simulink model "H_Full_Bridge_Inverter"  (R2023b)
settings: Solver=FixedStepDiscrete  StartTime=0.0  StopTime=0.1  FixedStep=10e-6  RelTol=1e-3
libraries: spsIGBTDiodeLib x4, simulink x1, spsCurrentMeasurementLib x1, spsDCVoltageSourceLib x1, spsSeriesRLCBranchLib x1, spsVoltageMeasurementLib x1, sps_lib x1
settings Model: Creator=aoni5  LastModifiedBy=aoni5

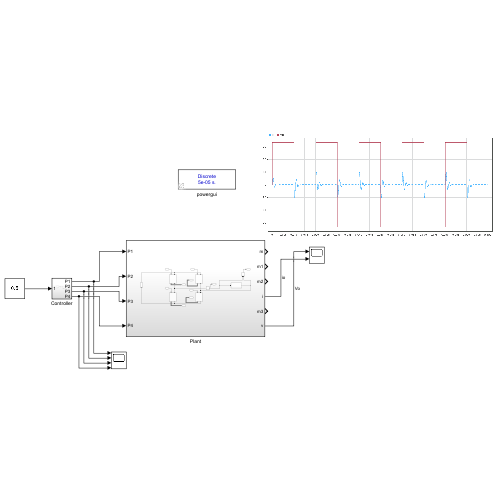
[thumbnail: Simulink's stored preview of the top-level diagram]
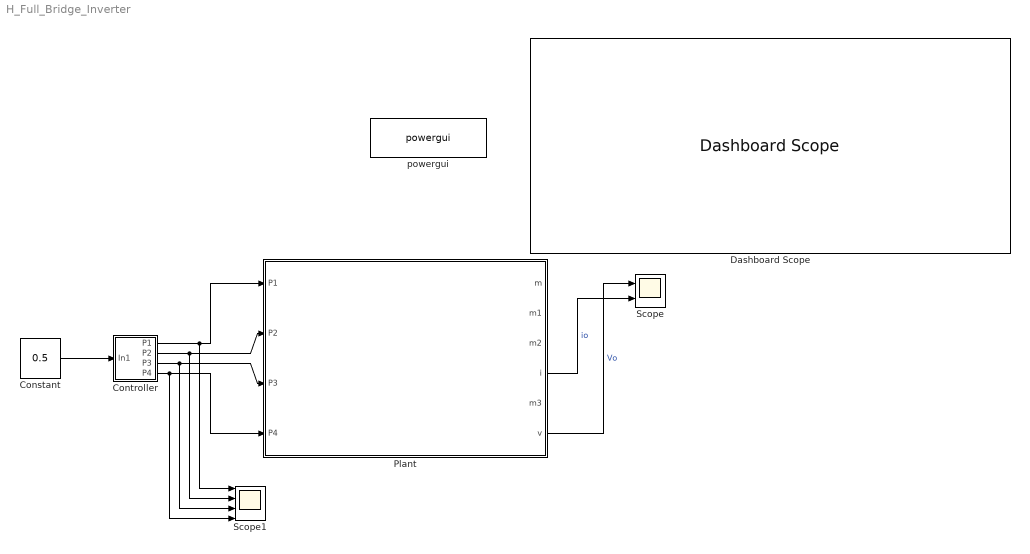
== system H_Full_Bridge_Inverter ==
  Constant : Constant  Value=0.5  VectorParams1D=off  SampleTime=50e-6
  Controller : Subsystem
  Dashboard Scope : DashboardScope
  Plant : Subsystem
  Scope : Scope  NumInputPorts=2
  Scope1 : Scope  NumInputPorts=4
  powergui : sps_lib/powergui  Priority=1  SimulationMode=Discrete  SampleTime=50e-6  frequency=60  Iterations=50  frequencyindice=0  Pbase=100e6  ErrMax=1e-4  UnitsV=kV  UnitsW=MW  buscounter=0  FunctionMessages=off  echomessages=off  EnableUseOfTLC=off  CurrentSourceSwitches=off  DisableSnubberDevices=off  DisableRonSwitches=off  DisableVfSwitches=off  DisplayEquations=off  AutomaticDiscreteSolvers=off  SolverType=Tustin/Backward Euler (TBE)  Interpol=off  ExternalGateDelay=off  methode=off  Ts=100  x0status=blocks  SPID=on  SwTol=0  HookPort=off  NonlinearTolerance=1e-4  nMaxIteration=100  ContinueOnMaxIteration=off  RestoreLinks=warning  ResistiveCurrentMeasurement=off  Frange=[0:2:500]  Ylog=off  Xlog=on  ShowGrid=off  save=off  variable=ZData  structure=0  ZoomFFT=off  StartTime=0.0  cycles=1  DisplayStyle=1  fundamental=60  FreqAxis=off  MaxFrequency=1000  frequencyindicesteady=1  RmsSteady=1  display=off
  wires:
  Constant/1 -> Controller/1(In1)
  Controller/1(P1) -> Scope1/1, Plant/1(P1)
  Plant/6(v) -> Scope/1  "Vo"
  Plant/4(i) -> Scope/2  "io"
  Controller/2(P2) -> Scope1/2, Plant/2(P2)
  Controller/3(P3) -> Scope1/3, Plant/3(P3)
  Controller/4(P4) -> Scope1/4, Plant/4(P4)

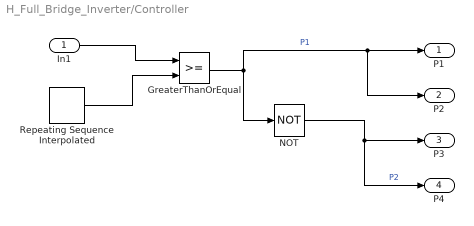
== system H_Full_Bridge_Inverter/Controller ==
  In1 : Inport
  GreaterThanOrEqual : RelationalOperator  OutDataTypeStr=boolean  RndMeth=Simplest  InputSameDT=off
  NOT : Logic  Operator=NOT  IconShape=distinctive  AllPortsSameDT=off  OutDataTypeStr=boolean
  Repeating Sequence Interpolated : simulink/Sources/Repeating Sequence Interpolated  OutValues=[0 1].'  TimeValues=[0 1/50].'  LookUpMeth=Interpolation-Use End Values  tsamp=50e-6  OutMin=[]  OutMax=[]  OutDataTypeStr=double  OutputDataTypeScalingMode=double  OutDataType=fixdt(0,8)  OutScaling=2^-10
  P1 : Outport
  P2 : Outport  Port=2
  P3 : Outport  Port=3
  P4 : Outport  Port=4
  wires:
  NOT/1 -> P4/1, P3/1  "P2"
  GreaterThanOrEqual/1 -> P2/1, P1/1, NOT/1  "P1"
  Repeating Sequence Interpolated/1 -> GreaterThanOrEqual/2
  In1/1 -> GreaterThanOrEqual/1

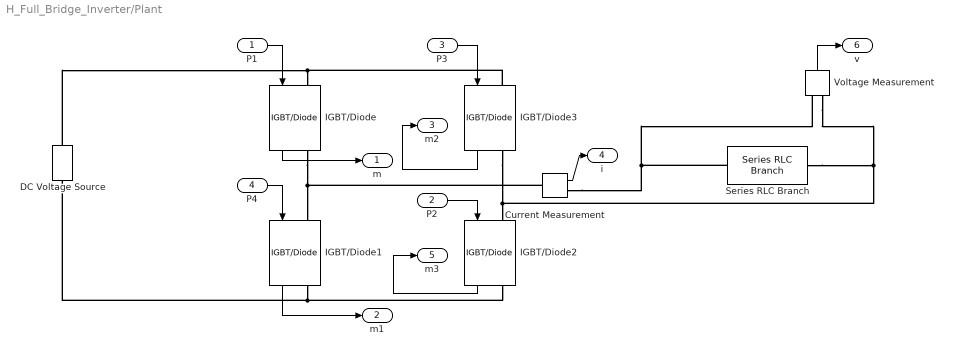
== system H_Full_Bridge_Inverter/Plant ==
  P1 : Inport
  P2 : Inport  Port=2
  P3 : Inport  Port=3
  P4 : Inport  Port=4
  Current Measurement : spsCurrentMeasurementLib/Current Measurement  PhasorSimulation=off  OutputType=Complex  PSBequivalent=0
  DC Voltage Source : spsDCVoltageSourceLib/DC Voltage Source  Amplitude=100  Measurements=None
  IGBT/Diode{,1..3} (4 alike) : spsIGBTDiodeLib/IGBT//Diode  Ron=1e-3  Rs=1e5  Cs=inf  Measurements=on
  Series RLC Branch : spsSeriesRLCBranchLib/Series RLC Branch  LConnTagsString=__new0  RConnTagsString=__new0  BranchType=RLC  Resistance=2.5  Inductance=1e-3  SetiL0=off  InitialCurrent=0  Capacitance=50e-6  Setx0=off  InitialVoltage=0  Measurements=None
  Voltage Measurement : spsVoltageMeasurementLib/Voltage Measurement  PhasorSimulation=off  OutputType=Complex  PSBequivalent=0
  m : Outport
  m1 : Outport  Port=2
  m2 : Outport  Port=3
  i : Outport  Port=4
  m3 : Outport  Port=5
  v : Outport  Port=6
  wires:
  P4/1 -> IGBT/Diode1/1
  P1/1 -> IGBT/Diode/1
  Voltage Measurement/1 -> v/1
  IGBT/Diode/1 -> m/1
  Current Measurement/1 -> i/1
  IGBT/Diode1/1 -> m1/1
  P2/1 -> IGBT/Diode2/1
  P3/1 -> IGBT/Diode3/1
  IGBT/Diode3/1 -> m2/1
  IGBT/Diode2/1 -> m3/1
  connections:
  IGBT/Diode1/RConn1 -- IGBT/Diode2/RConn1 -- DC Voltage Source/LConn1
  IGBT/Diode/RConn1 -- IGBT/Diode1/LConn1 -- Current Measurement/LConn1
  DC Voltage Source/RConn1 -- IGBT/Diode3/LConn1 -- IGBT/Diode/LConn1
  Series RLC Branch/LConn1 -- Voltage Measurement/LConn1 -- Current Measurement/RConn1
  Series RLC Branch/RConn1 -- Voltage Measurement/LConn2 -- IGBT/Diode2/LConn1 -- IGBT/Diode3/RConn1
